simulink model "pwm_avg_pred_controlled_system"  (R2017a)
settings: Solver=VariableStepAuto  StartTime=0.0  StopTime=t_f  RelTol=1e-3
values from neighbouring files (symbols this model uses):
  A = double(subs(A, symbs, vals))    [load_params.m]    (also in main.m)
  B = double(subs(B, symbs, vals))    [load_params.m]    (also in main.m)
  C = sysd.c    [load_discrete_pred_controller.m]    (also in load_params.m = double(subs(C, symbs, vals)); load_pwm_avg_pred_controller.m; main.m = double(subs(C, symbs, vals)))
  step_ref = torque_ref    [sim_controlled_system.m]
  Ts_val = 1.1e-2    (= 0.011)    [ss_value.m]
  x0 = [0; 0; 0]    [main.m]    (also in sim_controlled_system.m = [0; 0]; sim_system.m)
undefined symbols (not defined in the file or in its folder): Ctilde, Vcc_val
settings Model: Creator=brunolnetto  LastModifiedBy=brunolnetto
settings SolverCC: AlgebraicLoopSolver=LineSearch

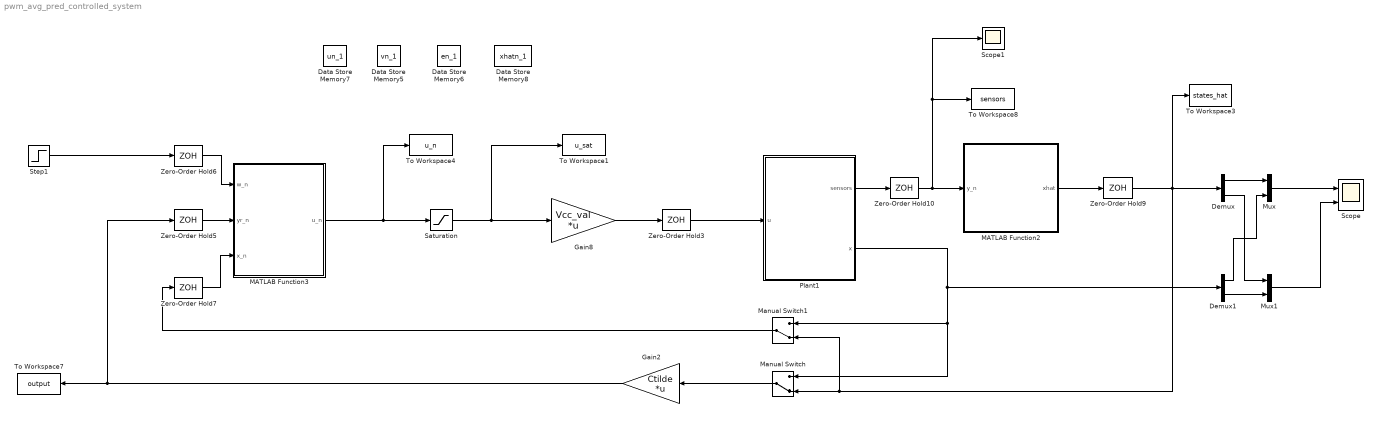
== system pwm_avg_pred_controlled_system ==
  Data Store Memory5 : DataStoreMemory  DataStoreName=vn_1  ReadBeforeWriteMsg=warning  WriteAfterWriteMsg=warning  WriteAfterReadMsg=warning  ShowAdditionalParam=off  OutDataTypeStr=double
  Data Store Memory6 : DataStoreMemory  DataStoreName=en_1  ReadBeforeWriteMsg=warning  WriteAfterWriteMsg=warning  WriteAfterReadMsg=warning  InitialValue=e0  ShowAdditionalParam=off  OutDataTypeStr=double
  Data Store Memory7 : DataStoreMemory  DataStoreName=un_1  ReadBeforeWriteMsg=warning  WriteAfterWriteMsg=warning  WriteAfterReadMsg=warning  ShowAdditionalParam=off  OutDataTypeStr=double
  Data Store Memory8 : DataStoreMemory  DataStoreName=xhatn_1  ReadBeforeWriteMsg=warning  WriteAfterWriteMsg=warning  WriteAfterReadMsg=warning  InitialValue=xhat0  ShowAdditionalParam=off  OutDataTypeStr=double
  Demux : Demux  Outputs=2
  Demux1 : Demux  Outputs=2
  Gain2 : Gain  Gain=Ctilde  Multiplication=Matrix(K*u) (u vector)
  Gain8 : Gain  Gain=Vcc_val  Multiplication=Matrix(K*u) (u vector)
  MATLAB Function2 : MATLAB Function  TreatAsAtomicUnit=on
  MATLAB Function3 : MATLAB Function  TreatAsAtomicUnit=on
  Manual Switch : ManualSwitch  CurrentSetting=0
  Manual Switch1 : ManualSwitch  CurrentSetting=0
  Mux : Mux  Inputs=2
  Mux1 : Mux  Inputs=2
  Plant1 : Subsystem
  Saturation : Saturate  UpperLimit=1  LowerLimit=-1
  Scope : Scope  NumInputPorts=2
  Scope1 : Scope
  Step1 : Step  Time=0  After=step_ref  SampleTime=Ts_val
  To Workspace1 : ToWorkspace  VariableName=u_sat  SaveFormat=Structure With Time  SampleTime=-1
  To Workspace3 : ToWorkspace  VariableName=states_hat  SaveFormat=Structure With Time  SampleTime=-1
  To Workspace4 : ToWorkspace  VariableName=u_n  SaveFormat=Structure With Time  SampleTime=-1
  To Workspace7 : ToWorkspace  VariableName=output  SaveFormat=Structure With Time  SampleTime=-1
  To Workspace8 : ToWorkspace  VariableName=sensors  SaveFormat=Structure With Time  SampleTime=-1
  Zero-Order Hold{3,5..7,9..10} (6 alike) : ZeroOrderHold  SampleTime=Ts_val
  wires:
  Mux/1 -> Scope/1
  Manual Switch1/1 -> Zero-Order Hold7/1
  Plant1/2(x) -> Manual Switch1/1, Manual Switch/1, Demux1/1
  Zero-Order Hold3/1 -> Plant1/1(u)
  Zero-Order Hold7/1 -> MATLAB Function3/3(x_n)
  Zero-Order Hold10/1 -> Scope1/1, To Workspace8/1, MATLAB Function2/1(y_n)
  Zero-Order Hold9/1 -> Demux/1, Manual Switch1/2, Manual Switch/2, To Workspace3/1
  Zero-Order Hold5/1 -> MATLAB Function3/2(yr_n)
  Gain2/1 -> Zero-Order Hold5/1, To Workspace7/1
  Plant1/1(sensors) -> Zero-Order Hold10/1
  Zero-Order Hold6/1 -> MATLAB Function3/1(w_n)
  Step1/1 -> Zero-Order Hold6/1
  Demux1/2 -> Mux1/2
  Demux1/1 -> Mux/2
  Mux1/1 -> Scope/2
  Manual Switch/1 -> Gain2/1
  Demux/2 -> Mux1/1
  Demux/1 -> Mux/1
  MATLAB Function2/1(xhat) -> Zero-Order Hold9/1
  Gain8/1 -> Zero-Order Hold3/1
  Saturation/1 -> To Workspace1/1, Gain8/1
  MATLAB Function3/1(u_n) -> To Workspace4/1, Saturation/1

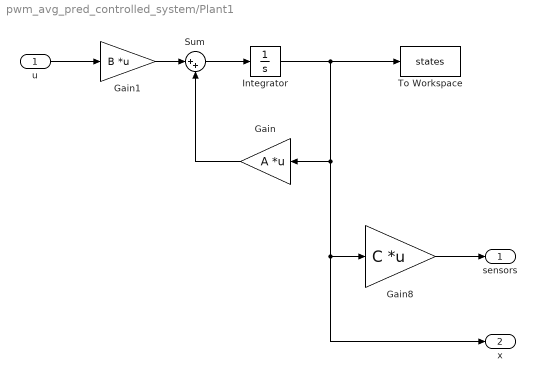
== system pwm_avg_pred_controlled_system/Plant1 ==
  u : Inport
  Gain : Gain  Gain=A  Multiplication=Matrix(K*u) (u vector)
  Gain1 : Gain  Gain=B  Multiplication=Matrix(K*u) (u vector)
  Gain8 : Gain  Gain=C  Multiplication=Matrix(K*u) (u vector)
  Integrator : Integrator  InitialCondition=x0
  Sum : Sum  Inputs=|++
  To Workspace : ToWorkspace  VariableName=states  SaveFormat=Structure With Time  SampleTime=-1
  sensors : Outport
  x : Outport  Port=2
  wires:
  Gain8/1 -> sensors/1
  Gain1/1 -> Sum/1
  u/1 -> Gain1/1
  Gain/1 -> Sum/2
  Sum/1 -> Integrator/1
  Integrator/1 -> To Workspace/1, x/1, Gain8/1, Gain/1

== matlab function pwm_avg_pred_controlled_system/MATLAB Function2 ==
  data: y_n input; xhat output; un_1 data_store_memory; xhatn_1 data_store_memory; params parameter
function xhat = observador (y_n, params)
    global un_1;
    global xhatn_1;
    
%     x_bar = params.Phi*xhatn_1 + params.Gamma*un_1;
%     xhat = x_bar + params.L*(y - params.C*xhatn_1);
    
    Phi = params.Phi;
    Gamma = params.Gamma;
    L = params.L;
    C = params.C;

    xhat = Phi*xhatn_1 + Gamma*un_1 + L*(y_n - C*xhatn_1);

    xhatn_1 = xhat;
end

== matlab function pwm_avg_pred_controlled_system/MATLAB Function3 ==
  data: w_n input; yr_n input; x_n input; u_n output; vn_1 data_store_memory; params parameter; en_1 data_store_memory; un_1 data_store_memory
function u_n = controller(w_n, yr_n, x_n, params)
    global vn_1;
    global en_1;
    global un_1;
    
    v_n = vn_1 + en_1;
    
    u_i = params.Ki*v_n;
    u_p = - params.Kp*x_n;
    
    u_n = u_i + u_p;
    
    vn_1 = v_n;
    en_1 = w_n - yr_n;
    un_1 = u_n;
end
